simulink model "arduino_ros_matlab"  (R2022b)
settings: Solver=VariableStepAuto  StartTime=0.0  StopTime=inf  RelTol=1e-3
libraries: robotlib x4
settings Model: Creator=genis  LastModifiedBy=genis

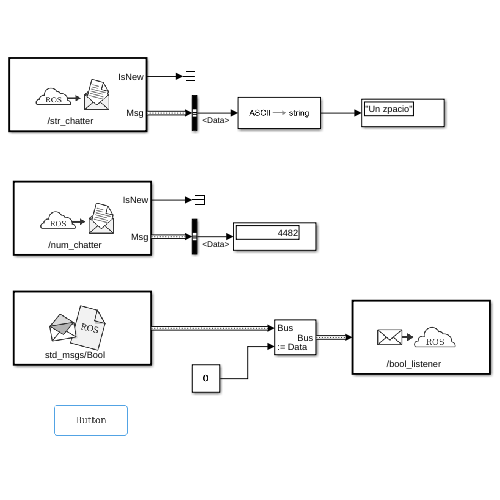
[thumbnail: Simulink's stored preview of the top-level diagram]
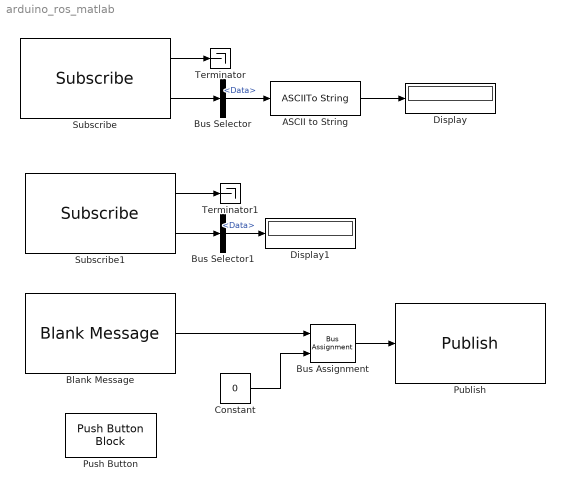
== system arduino_ros_matlab ==
  ASCII to String : ASCIIToString
  Blank Message : robotlib/Blank Message  messageClass=Message  entityType=std_msgs/Bool  messageType=std_msgs/Bool  SampleTime=inf  legacyBusStruct=off
      settings: LibrarySourceBlock=roslib/ROS/Blank Message
  Bus Assignment : BusAssignment  AssignedSignals=Data
  Bus Selector : BusSelector  OutputSignals=Data
  Bus Selector1 : BusSelector  OutputSignals=Data
  Constant : Constant  Value=0  OutDataTypeStr=boolean
  Display : Display
  Display1 : Display
  Publish : robotlib/Publish  topicSource=Select from ROS network  topic=/bool_listener  messageType=std_msgs/Bool  legacyBusStruct=off  messageQueueLength=1
      settings: LibrarySourceBlock=roslib/ROS/Publish
  Push Button : PushButtonBlock  ButtonType=Latch  OffValue=0.000000
  Subscribe : robotlib/Subscribe  topicSource=Select from ROS network  topic=/str_chatter  messageType=std_msgs/String  SampleTime=-1  legacyBusStruct=off  messageQueueLength=1
      settings: LibrarySourceBlock=roslib/ROS/Subscribe
  Subscribe1 : robotlib/Subscribe  topicSource=Select from ROS network  topic=/num_chatter  messageType=std_msgs/Int32  SampleTime=-1  legacyBusStruct=off  messageQueueLength=1
      settings: LibrarySourceBlock=roslib/ROS/Subscribe
  Terminator : Terminator
  Terminator1 : Terminator
  wires:
  Subscribe/1 -> Terminator/1
  Subscribe/2 -> Bus Selector/1
  ASCII to String/1 -> Display/1
  Bus Selector/1 -> ASCII to String/1  "<Data>"
  Subscribe1/1 -> Terminator1/1
  Bus Selector1/1 -> Display1/1  "<Data>"
  Subscribe1/2 -> Bus Selector1/1
  Blank Message/1 -> Bus Assignment/1
  Constant/1 -> Bus Assignment/2
  Bus Assignment/1 -> Publish/1
